simulink model "controle2_observador"  (R2023b)
settings: Solver=ode45  StartTime=0.0  StopTime=20  RelTol=1e-3  EnableMultiTasking=on
values from neighbouring files (symbols this model uses):
  A = [ ... (first row only)    [controle2.m]
  B = [ ... (first row only)    [controle2.m]
  C = [1.0     0.0     0.0     0.0]    [controle2.m]
  Ka = Kt(1:4)    [controle2.m]
  Ki = -Kt(5)    [controle2.m]
  L = L'    [controle2.m]
settings Model: Creator=LENOVO  LastModifiedBy=mluser
settings SolverCC: AlgebraicLoopSolver=TrustRegion
settings DataIOCC: LimitDataPoints=on  SaveFormat=Array  ReturnWorkspaceOutputs=off
settings OptimizationCC: LifeSpan=inf
settings DebuggingCC: UnconnectedInputMsg=warning  UnconnectedOutputMsg=warning  UnconnectedLineMsg=warning  SFUnexpectedBacktrackingDiag=warning  SFNoUnconditionalDefaultTransitionDiag=warning  SFExecutionAtInitializationDiag=none  ArithmeticOperatorsInVariantConditions=warning
settings HardwareCC: ProdBitPerPointer=32  ProdBitPerSizeT=32  ProdBitPerPtrDiffT=32  ProdLargestAtomicFloat=None  ProdIntDivRoundTo=Undefined  ProdEndianess=Unspecified  ProdWordSize=32  ProdHWDeviceType=32-bit Generic
settings ModelReferenceCC: EnableRefExpFcnMdlSchedulingChecks=on  PropagateSignalLabelsOutOfModel=off
settings SFSimCC: SimUseLocalCustomCode=off  CustomCodeUndefinedFunction=UseInterfaceOnly
settings RTWCC: RTWUseLocalCustomCode=off  DLArmComputeVersion=19.05
settings CodeAppCC: StateflowObjectComments=on
settings GRTTargetCC: TargetLangStandard=C89/C90 (ANSI)
settings ConfigComp: CovMetricSettings=dw  CovSaveCumulativeToWorkspaceVar=on  CovSaveSingleToWorkspaceVar=on  CovExternalEMLEnable=off

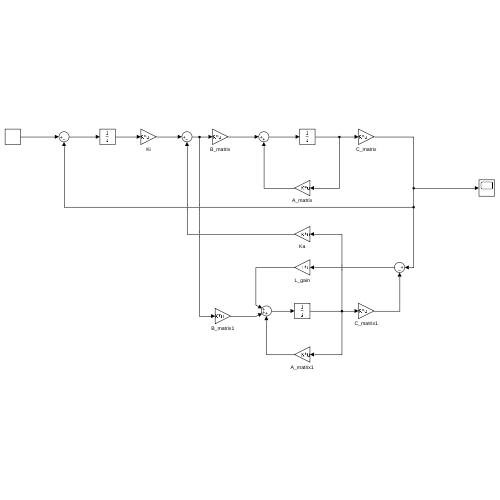
[thumbnail: Simulink's stored preview of the top-level diagram]
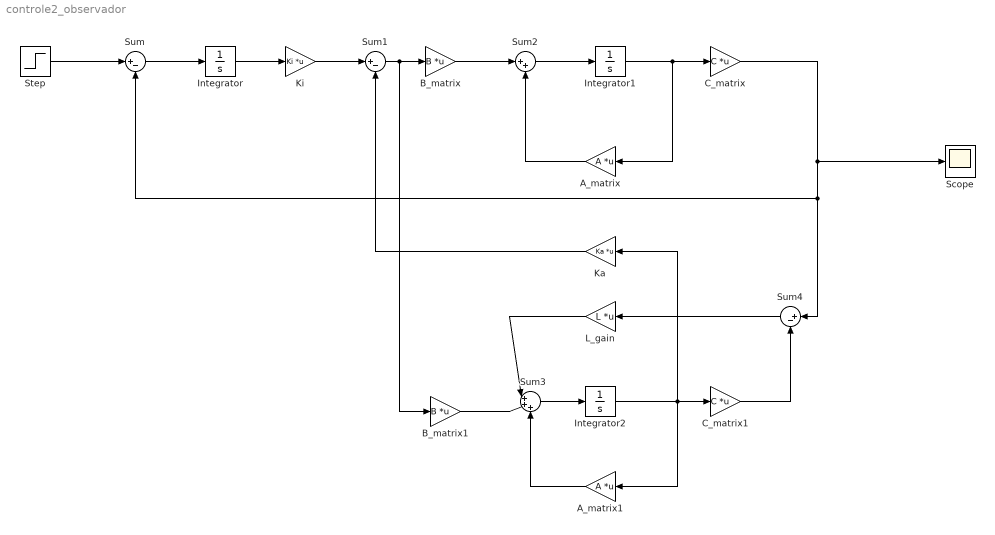
== system controle2_observador ==
  A_matrix : Gain  Gain=A  Multiplication=Matrix(K*u)
  A_matrix1 : Gain  Gain=A  Multiplication=Matrix(K*u)
  B_matrix : Gain  Gain=B  Multiplication=Matrix(K*u)
  B_matrix1 : Gain  Gain=B  Multiplication=Matrix(K*u)
  C_matrix : Gain  Gain=C  Multiplication=Matrix(K*u)
  C_matrix1 : Gain  Gain=C  Multiplication=Matrix(K*u)
  Integrator : Integrator
  Integrator1 : Integrator
  Integrator2 : Integrator
  Ka : Gain  Gain=Ka  Multiplication=Matrix(K*u)
  Ki : Gain  Gain=Ki  Multiplication=Matrix(K*u)
  L_gain : Gain  Gain=L  Multiplication=Matrix(K*u)
  Scope : Scope
  Step : Step  Time=0  SampleTime=20
  Sum : Sum  Inputs=|+-
  Sum1 : Sum  Inputs=|+-
  Sum2 : Sum  Inputs=|++
  Sum3 : Sum  Inputs=|+++
  Sum4 : Sum  Inputs=|+-
  wires:
  Sum/1 -> Integrator/1
  Integrator/1 -> Ki/1
  Ki/1 -> Sum1/1
  Step/1 -> Sum/1
  Sum1/1 -> B_matrix1/1, B_matrix/1
  B_matrix/1 -> Sum2/1
  Sum2/1 -> Integrator1/1
  Integrator1/1 -> A_matrix/1, C_matrix/1
  A_matrix/1 -> Sum2/2
  Ka/1 -> Sum1/2
  Sum3/1 -> Integrator2/1
  Integrator2/1 -> A_matrix1/1, C_matrix1/1, Ka/1
  A_matrix1/1 -> Sum3/3
  B_matrix1/1 -> Sum3/2
  C_matrix1/1 -> Sum4/2
  Sum4/1 -> L_gain/1
  L_gain/1 -> Sum3/1
  C_matrix/1 -> Scope/1, Sum4/1, Sum/2
